simulink model "Reference_model_Control_Engineering"  (R2021b)
settings: Solver=FixedStepDiscrete  StartTime=0.0  StopTime=inf  FixedStep=Ts  RelTol=1e-3  EnableMultiTasking=on
InitFcn:
  | Fs = 4000; Ts = 1/Fs; tsim = 29.9997;
libraries: sperte_lib x116
settings Model: SimulationMode=external  Creator=Enzo  LastModifiedBy=20191981
settings SolverCC: AlgebraicLoopSolver=TrustRegion  PositivePriorityOrder=on
settings DataIOCC: SaveOutput=off  DSMLogging=off  SaveTime=off  ReturnWorkspaceOutputs=off
settings OptimizationCC: EnhancedBackFolding=on  PassReuseOutputArgsThreshold=0  MaxStackSize=64  OptimizeBlockOrder=speed  DifferentSizesBufferReuse=on  OptimizationCustomize=off
settings DebuggingCC: ParameterTunabilityLossMsg=error  SFMachineParentedDataDiag=warning  ArithmeticOperatorsInVariantConditions=warning
settings HardwareCC: ProdBitPerPointer=32  ProdBitPerSizeT=32  ProdBitPerPtrDiffT=32  ProdLargestAtomicInteger=Long  ProdLargestAtomicFloat=Double  ProdWordSize=32  ProdLongLongMode=on  ProdHWDeviceType=ARM Compatible->ARM Cortex  UseEmbeddedCoderFeatures=off
settings SFSimCC: CustomCodeUndefinedFunction=UseInterfaceOnly
settings RTWCC: Description=Embedded Coder  SystemTargetFile=ert.tlc  HardwareBoard=Raspberry Pi  TLCOptions="-aInlineSetEventsForThisBaseRateFcn=TLC_FALSE -aSuppressMultiTaskScheduler=TLC_FALSE  -aRateBasedStepFcn=0"  TemplateMakefile=ert_default_tmf  PostCodeGenCommand="if (~verLessThan('matlab', '9.11')) codertarget.postCodeGenHookCommand(h);  SPERTE_postGenFunc(modelName, buildInfo); else; SPERTE_postGenFunc(h, buildInfo); end"  Toolchain=GNU GCC Embedded Linux  BuildConfiguration=Faster Runs
settings CodeAppCC: ForceParamTrailComments=on  OperatorAnnotations=on
settings ERTTargetCC: ERTCustomFileBanners=off  SupportContinuousTime=on  SupportNonInlinedSFcns=on  RemoveResetFunc=off  SupportVariableSizeSignals=on  ModelStepFunctionPrototypeControlCompliant=off  ExtMode=on  ExtModeMexArgs='sperte0.bwk.tue.nl' 0 17725  ERTSrcFileBannerTemplate=codertarget_code_template.cgt  ERTHdrFileBannerTemplate=codertarget_code_template.cgt  ERTDataSrcFileTemplate=codertarget_code_template.cgt  ERTDataHdrFileTemplate=codertarget_code_template.cgt

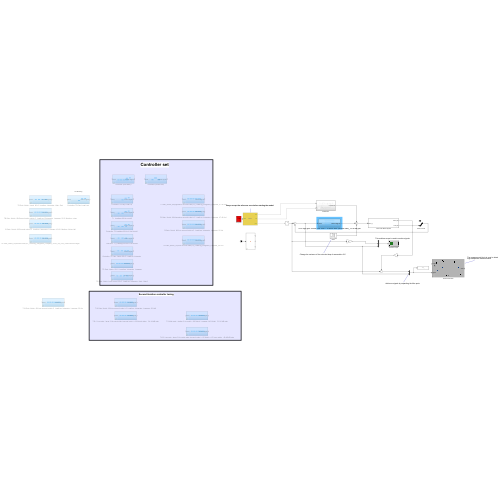
[thumbnail: Simulink's stored preview of the top-level diagram]
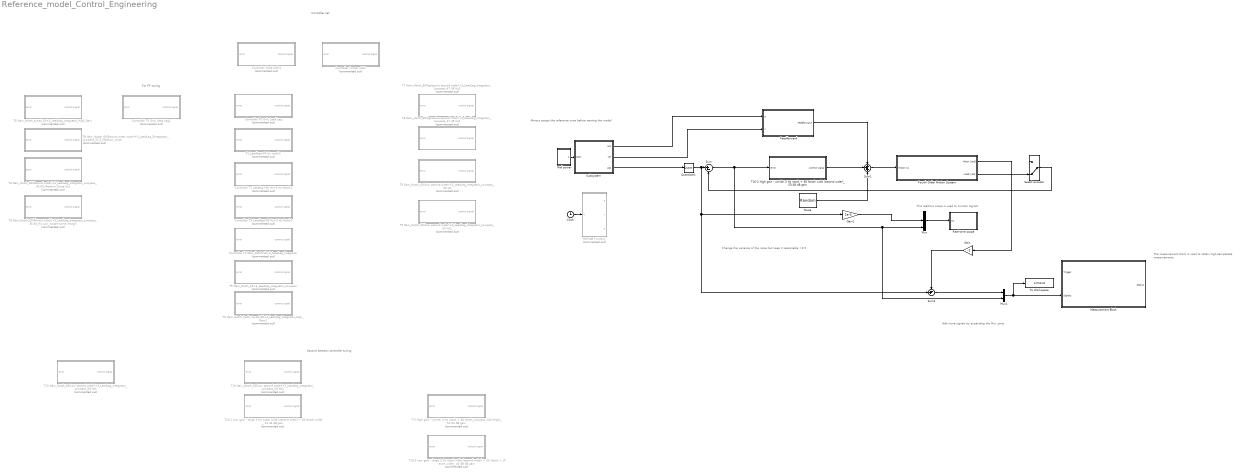
== system Reference_model_Control_Engineering ==
  note: Add more signals by expanding the Mux ports
  note: The measurement block is used to obtain high-samplerate measurements
  note: This realtime scope is used to monitor signals
  note: Always accept the reference once before starting the model.
  note: Change the variance of the noise but keep it reasonable <0.5
  note: Second iteration controller tuning
  note: For FF tuning
  note: Controller set
  Clock : Clock
  Controller (load side)1 : Subsystem  Commented=on
  Controller (motor side) : Subsystem  Commented=on
  Controller T0 Only Lead Lag : Subsystem  Commented=on
  Controller T0 Only Lead Lag1 : Subsystem  Commented=on
  Controller T2 Leadlag+60 Hz+3 Hz Notch1 : Subsystem  Commented=on
  Controller T3_Leadlag+60 Hz+3 Hz Notch1 : Subsystem  Commented=on
  Controller T4 Gain_Notch 60+3_LeadLag_Integrator : Subsystem  Commented=on
  Feedforward : Subsystem
  Fourth Order Motion System : Subsystem
  Gain : Gain  Gain=-1
  Gain1 : Gain  Gain=1e-3
  MATLAB Function : MATLAB Function  Commented=on  TreatAsAtomicUnit=on
  Measurement Block : Subsystem  Description=|  Priority=-1  mask(SPERTE Lib){N_samples=300000, triggertype=2, trigger_command=0}
      | Perform on-demand measurements to file using this block.
      | 
      | It can be used in 2 ways:
      | 1) Set the mask triggertype parameter to manual and use the trigger input signal to trigger a measurement.
      | You can do this by providing a 0 to 1 transition.
      | Keep it low after you start/complete the measurement, or it will measure again.
      | A file is created with measurement_0,1,2... etc
      | 
      | 2) Keep the model running, and trigger a measurement from the commandline or Matlab script.
      | For example:
      | 
      | % How many samples to measure?
      | N_samples = Fs*5;
      | % Do the measurement
      | SPERTE_Perform_Measurement(N_samples);
      | % Get the latest file
      | file_list = SPERTE_Get_Latest_Measurement(p,1,'./data');
      | % How many signals did you record?
      | N_signals = 3;
      | % Convert the .bin to .mat and return the results
      | measurement = SPERTE_Bin_To_Mat(file_list,N_signals);
      mask prompts: N_samples "Number of samples"; trigger_command "Trigger command"
      mask help:
      | This block implements a measurement to file sink.
      | It can be used in two ways:
      | 1) Triggered from the simulink model
      | 2) Triggered from the command line
      mask Help:
      | Perform on-demand measurements to file using this block.
      | 
      | It can be used in 2 ways:
      | 1) Set the mask triggertype parameter to manual and use the trigger input signal to trigger a measurement.
      | You can do this by providing a 0 to 1 transition.
      | Keep it low after you start/complete the measurement, or it will measure again.
      | A file is created with measurement_0,1,2... etc
      | 
      | 2) Keep the model running, and trigger a measurement from the commandline or Matlab script.
      | For example:
      | 
      | % How many samples to measure?
      | N_samples = Fs*5;
      | % Do the measurement
      | SPERTE_Perform_Measurement(N_samples);
      | % Get the latest file
      | file_list = SPERTE_Get_Latest_Measurement(p,1,'./data');
      | % How many signals did you record?
      | N_signals = 3;
      | % Convert the .bin to .mat and return the results
      | measurement = SPERTE_Bin_To_Mat(file_list,N_signals);
      mask TypeOptions N_samples: SPERTE_measurement_samples/Value
      mask TypeOptions trigger_command: SPERTE_measurement_trigger_command/Value
      mask DialogControl BlockName Prompt: Sperte measurement block.
      mask DialogControl Desc Prompt: Can be used to trace signals to .bin file on the Raspberry Pi.  Can be triggered through signals in the simulink model or manually.
      mask DialogControl TriggerText Prompt: Manual (0), Command (1), Both (2)
      mask Display: ud = get_param(gcb,'UserData');image(ud.x);
  Mux : Mux  Inputs=3
  Mux1 : Mux  Inputs=2
  Noise : RandomNumber  Variance=0  SampleTime=Ts
  Quantizer1 : Quantizer  QuantizationInterval=(2*pi)/(500*4)
  Real-time scope : Subsystem  Priority=0  mask(Scope){Sample_Time=1/500}
      mask prompts: Sample_Time "Scope sample time"
      mask help:
      | Realtime Scope block allows one to view the signals while the model is running.
      | The signals are downsampled to a specified sample rate (in the mask parameter) to reduce communication overhead.
      settings: CopyFcn=set_param(gcb,'LinkStatus','None')  OpenFcn=open_system(strcat(get_param(gcb,'Parent'),'/',get_param(gcb,'Name'),'/Live_Scope'),'force');
      mask TypeOptions Sample_Time: Downsample/OutPortSampleTime
      mask DialogControl scopebutton Prompt: Open the live scope
      mask DialogControl scopebutton Callback: open_system(strcat(get_param(gcb,'Parent'),'/',get_param(gcb,'Name'),'/Live_Scope'));
      mask Display: ud = get_param(gcb,'UserData');image(ud.x);
  Ref power : Subsystem  mask(On/Off Switch){stat=On}
      mask prompts: stat "Switch"
      mask TypeOptions stat: On | Off
  Select encoder : ManualSwitch  CurrentSetting=0
  Subsystem : Subsystem  mask(Ref3){}
      settings: OpenFcn=global ref_part; cb_axes 1
      mask Display: disp('Ref3');
  Sum : Sum  Inputs=|+-
  Sum1 : Sum  Inputs=+++
  Sum2 : Sum  Inputs=-+|
  T-II High gain - similar 3 Hz notch + 60 Notch_Lowpass 140 (High)_ 51.04 dB gain : Subsystem  Commented=on
  T10 Gain_Notch_60(Low second order)+3_LeadLag_Integrator_Lowpass_50 Hz1 : Subsystem  Commented=on
  T10 Gain_Notch_60(Low second order)+3_LeadLag_Integrator_Lowpass_50 Hz2 : Subsystem  Commented=on
  T10-1 Low gain - large 3 Hz notch wide (second order) + 60 Notch wider _ 24.44 dB gain : Subsystem  Commented=on
  T10-2 High gain - similar 3 Hz notch + 60 Notch wide (second order)_ 53.68 dB gain : Subsystem
  T10-3 Low gain - large 3 Hz notch wide (second order) + 60 Notch + LP even wider_ 40 dB dB gain : Subsystem  Commented=on
  T1_Leadlag+60 Hz notch2 : Subsystem  Commented=on
  T5 Gain_Notch_60+3_LeadLag_Integrator_Lowpass : Subsystem  Commented=on
  T5 Gain_Notch_tuned_60+3_LeadLag_Integrator_High_Gain : Subsystem  Commented=on
  T6 Gain_Notch_badly tuned_60+3_LeadLag_Integrator_High_Gain2 : Subsystem  Commented=on
  T7 Gain_Notch_60(Agressive second order)+3_LeadLag_Integrator_Lowpass_47.49 Hz2 : Subsystem  Commented=on
  T8 Gain_Notch_60(Agressive second order)+3_LeadLag_Integrator_Lowpass_47.49 Hz1 : Subsystem  Commented=on
  T8 Gain_Notch_60(Almost notch)+3_LeadLag_Integrator_Lowpass_35.60_Hz_Low_noise+some margin : Subsystem  Commented=on
  T9 Gain_Notch_60(Low second order)+3_LeadLag_Integrator_Lowpass_50 Hz : Subsystem  Commented=on
  T9 Gain_Notch_60(Low second order)+3_LeadLag_Integrator_Lowpass_50 Hz1 : Subsystem  Commented=on
  TA Gain_Notch_60(Second order)+3_LeadLag_Integrator_Lowpass_43.69_Medium_Noise Hz1 : Subsystem  Commented=on
  TB Gain_Notch_60(Second order notch)+3_LeadLag_DIntegrator_Lowpass_52.5_Medium_noise : Subsystem  Commented=on
  To Workspace : ToWorkspace  VariableName=simout  SampleTime=-1
  wires:
  Select encoder/1 -> Sum/2
  Sum1/1 -> Fourth Order Motion System/1(Motor [v])
  Sum/1 -> T10-2 High gain - similar 3 Hz notch + 60 Notch wide (second order)_ 53.68 dB gain/1(error), Mux1/2, Mux/3
  Quantizer1/1 -> Sum2/2, Gain1/1, Sum/1
  Ref power/1(On/Off) -> Subsystem/1(start)
  Mux/1 -> Real-time scope/1(In1)
  Noise/1 -> Sum1/3
  Mux1/1 -> To Workspace/1, Measurement Block/2(Signals)
  Clock/1 -> MATLAB Function/1(t)
  Feedforward/1(Feedforward) -> Sum1/1
  Gain/1 -> Sum2/1
  Subsystem/3(pos) -> Quantizer1/1
  Subsystem/2(vel) -> Feedforward/2(v)
  Subsystem/1(acc) -> Feedforward/1(a)
  Fourth Order Motion System/2(Load [rad]) -> Select encoder/2
  Fourth Order Motion System/1(Motor [rad]) -> Gain/1
  T10-2 High gain - similar 3 Hz notch + 60 Notch wide (second order)_ 53.68 dB gain/1(control signal) -> Sum1/2
  Gain1/1 -> Mux/2
  Sum2/1 -> Mux1/1

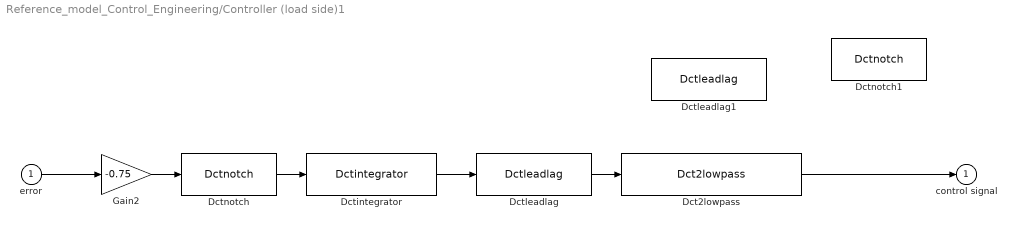
== system Reference_model_Control_Engineering/Controller (load side)1 ==
  error : Inport
  Dct2lowpass : sperte_lib/Dct2lowpass  f_den=60  b_den=0.075
      settings: SourceProductName=SPERTE project library
  Dctintegrator : sperte_lib/Dctintegrator  f_num=7.5
      settings: SourceProductName=SPERTE project library
  Dctleadlag : sperte_lib/Dctleadlag  f_num=4.5  f_den=1000
      settings: SourceProductName=SPERTE project library
  Dctleadlag1 : sperte_lib/Dctleadlag  f_num=5  f_den=50
      settings: SourceProductName=SPERTE project library
  Dctnotch : sperte_lib/Dctnotch  f_num=60.9  b_num=0.015  f_den=95  b_den=0.90
      settings: SourceProductName=SPERTE project library
  Dctnotch1 : sperte_lib/Dctnotch  f_num=2.6  b_num=0.3  f_den=2.6  b_den=0.001
      settings: SourceProductName=SPERTE project library
  Gain2 : Gain  Gain=-0.75
  control signal : Outport
  wires:
  error/1 -> Gain2/1
  Gain2/1 -> Dctnotch/1
  Dctnotch/1 -> Dctintegrator/1
  Dctintegrator/1 -> Dctleadlag/1
  Dctleadlag/1 -> Dct2lowpass/1
  Dct2lowpass/1 -> control signal/1

== system Reference_model_Control_Engineering/Controller (motor side) ==
  error : Inport
  Dctintegrator : sperte_lib/Dctintegrator  f_num=5
      settings: SourceProductName=SPERTE project library
  Dctleadlag : sperte_lib/Dctleadlag  f_num=6  f_den=130
      settings: SourceProductName=SPERTE project library
  Dctnotch : sperte_lib/Dctnotch  f_num=59  b_num=0.05  f_den=63  b_den=0.5
      settings: SourceProductName=SPERTE project library
  Gain2 : Gain  Gain=4.06
  control signal : Outport
  wires:
  error/1 -> Gain2/1
  Dctleadlag/1 -> control signal/1
  Gain2/1 -> Dctnotch/1
  Dctnotch/1 -> Dctleadlag/1

== system Reference_model_Control_Engineering/Controller T0 Only Lead Lag ==
  error : Inport
  Dctleadlag1 : sperte_lib/Dctleadlag  f_num=5  f_den=50
      settings: SourceProductName=SPERTE project library
  Dctnotch1 : sperte_lib/Dctnotch  f_num=2.6  b_num=0.3  f_den=2.6  b_den=0.001
      settings: SourceProductName=SPERTE project library
  Gain2 : Gain  Gain=-1
  Test_0_Dctleadlag : sperte_lib/Dctleadlag  f_num=6  f_den=17
      settings: SourceProductName=SPERTE project library
  control signal : Outport
  wires:
  error/1 -> Gain2/1
  Test_0_Dctleadlag/1 -> control signal/1
  Gain2/1 -> Test_0_Dctleadlag/1

== system Reference_model_Control_Engineering/Controller T0 Only Lead Lag1 ==
  error : Inport
  Dctleadlag1 : sperte_lib/Dctleadlag  f_num=5  f_den=50
      settings: SourceProductName=SPERTE project library
  Dctnotch1 : sperte_lib/Dctnotch  f_num=2.6  b_num=0.3  f_den=2.6  b_den=0.001
      settings: SourceProductName=SPERTE project library
  Gain2 : Gain  Gain=-1
  Test_0_Dctleadlag : sperte_lib/Dctleadlag  f_num=6  f_den=17
      settings: SourceProductName=SPERTE project library
  control signal : Outport
  wires:
  error/1 -> Gain2/1
  Test_0_Dctleadlag/1 -> control signal/1
  Gain2/1 -> Test_0_Dctleadlag/1

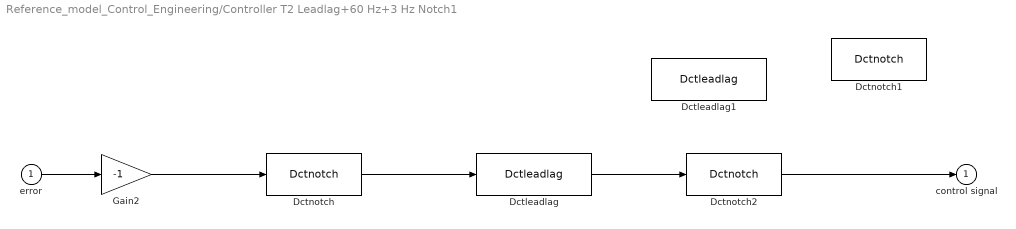
== system Reference_model_Control_Engineering/Controller T2 Leadlag+60 Hz+3 Hz Notch1 ==
  error : Inport
  Dctleadlag : sperte_lib/Dctleadlag  f_num=4.4195  f_den=180
      settings: SourceProductName=SPERTE project library
  Dctleadlag1 : sperte_lib/Dctleadlag  f_num=5  f_den=50
      settings: SourceProductName=SPERTE project library
  Dctnotch : sperte_lib/Dctnotch  f_num=60.95  b_num=0.01  f_den=60.95  b_den=0.6
      settings: SourceProductName=SPERTE project library
  Dctnotch1 : sperte_lib/Dctnotch  f_num=2.6  b_num=0.3  f_den=2.6  b_den=0.001
      settings: SourceProductName=SPERTE project library
  Dctnotch2 : sperte_lib/Dctnotch  f_num=3.25  b_num=0.5  f_den=3.25  b_den=0.025
      settings: SourceProductName=SPERTE project library
  Gain2 : Gain  Gain=-1
  control signal : Outport
  wires:
  error/1 -> Gain2/1
  Gain2/1 -> Dctnotch/1
  Dctleadlag/1 -> Dctnotch2/1
  Dctnotch/1 -> Dctleadlag/1
  Dctnotch2/1 -> control signal/1

== system Reference_model_Control_Engineering/Controller T3_Leadlag+60 Hz+3 Hz Notch1 ==
  error : Inport
  Dctleadlag : sperte_lib/Dctleadlag  f_num=5  f_den=400
      settings: SourceProductName=SPERTE project library
  Dctnotch : sperte_lib/Dctnotch  f_num=60.6  b_num=0.015  f_den=60.6  b_den=0.5
      settings: SourceProductName=SPERTE project library
  Dctnotch2 : sperte_lib/Dctnotch  f_num=3.25  b_num=0.5  f_den=3.25  b_den=0.025
      settings: SourceProductName=SPERTE project library
  Gain2 : Gain  Gain=-0.95
  control signal : Outport
  wires:
  error/1 -> Gain2/1
  Gain2/1 -> Dctnotch/1
  Dctleadlag/1 -> Dctnotch2/1
  Dctnotch/1 -> Dctleadlag/1
  Dctnotch2/1 -> control signal/1

== system Reference_model_Control_Engineering/Controller T4 Gain_Notch 60+3_LeadLag_Integrator ==
  error : Inport
  Dctintegrator : sperte_lib/Dctintegrator  f_num=7
      settings: SourceProductName=SPERTE project library
  Dctleadlag : sperte_lib/Dctleadlag  f_num=3.975  f_den=400
      settings: SourceProductName=SPERTE project library
  Dctnotch : sperte_lib/Dctnotch  f_num=60.6  b_num=0.015  f_den=90  b_den=0.5
      settings: SourceProductName=SPERTE project library
  Dctnotch2 : sperte_lib/Dctnotch  f_num=3.25  b_num=0.5  f_den=3.25  b_den=0.025
      settings: SourceProductName=SPERTE project library
  Gain2 : Gain  Gain=-0.95
  control signal : Outport
  wires:
  error/1 -> Gain2/1
  Gain2/1 -> Dctnotch/1
  Dctleadlag/1 -> Dctnotch2/1
  Dctnotch/1 -> Dctleadlag/1
  Dctnotch2/1 -> Dctintegrator/1
  Dctintegrator/1 -> control signal/1

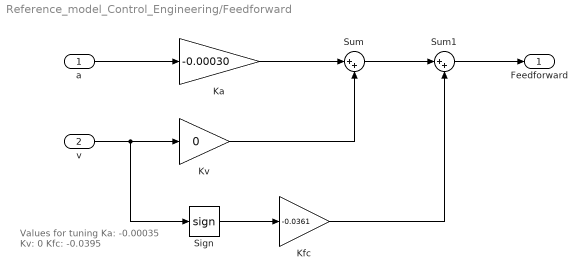
== system Reference_model_Control_Engineering/Feedforward ==
  note: Values for tuning
      | Ka: -0.00035
      | Kv: 	0
      | Kfc: -0.0395
  a : Inport
  v : Inport  Port=2
  Ka : Gain  Gain=-0.00030
  Kfc : Gain  Gain=-0.0361
  Kv : Gain  Gain=0
  Sign : Signum
  Sum : Sum  Inputs=|++
  Sum1 : Sum  Inputs=|++
  Feedforward : Outport
  wires:
  a/1 -> Ka/1
  Ka/1 -> Sum/1
  v/1 -> Sign/1, Kv/1
  Kv/1 -> Sum/2
  Sign/1 -> Kfc/1
  Sum/1 -> Sum1/1
  Kfc/1 -> Sum1/2
  Sum1/1 -> Feedforward/1

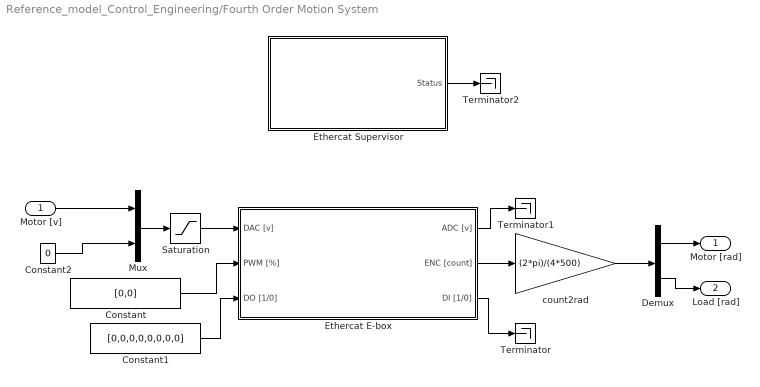
== system Reference_model_Control_Engineering/Fourth Order Motion System ==
  Motor [v] : Inport
  Constant : Constant  Value=[0,0]
  Constant1 : Constant  Value=[0,0,0,0,0,0,0,0]
  Constant2 : Constant  Value=0
  Demux : Demux  Outputs=2
  Ethercat E-box : Subsystem  Priority=-2  mask(Sperte Lib){link_id=0}
      mask prompts: link_id "Link ID of the specific ebox"
      mask help:
      | This block implements a single E-box device.
      | Ensure that if you have multiple E-box devices that they each have an unique link_id.
      |
      | You MUST have an Ethercat Initialize block in your model to be able to use this block.
      mask Display: ud = get_param(gcb,'UserData');image(ud.x);
  Ethercat Supervisor : Subsystem  Description=Must be executed first, keep at -1 priority (highest)  Priority=-3  mask(Sperte Lib){portid=0, ectimeout=500}
      mask prompts: portid "Ethernet port number for the Ethercat protocol (default 0 = eth0)"; ectimeout "Timeout of the Ethercat protocol in microseconds."
      mask help:
      | This block initializes the Ethercat connection on the Raspberry Pi.
      |
      | This enables you to use multiple E-box devices by including multiple blocks of the "Ethercat E-box" type.
      mask Display: ud = get_param(gcb,'UserData');image(ud.x);
  Mux : Mux  Inputs=2
  Saturation : Saturate  UpperLimit=2.5  LowerLimit=-2.5
  Terminator : Terminator
  Terminator1 : Terminator
  Terminator2 : Terminator
  count2rad : Gain  Gain=(2*pi)/(4*500)
  Motor [rad] : Outport
  Load [rad] : Outport  Port=2
  wires:
  Ethercat E-box/1(ADC [v]) -> Terminator1/1
  Ethercat E-box/2(ENC [count]) -> count2rad/1
  Constant/1 -> Ethercat E-box/2(PWM [%])
  Mux/1 -> Saturation/1
  count2rad/1 -> Demux/1
  Motor [v]/1 -> Mux/1
  Constant2/1 -> Mux/2
  Demux/1 -> Motor [rad]/1
  Demux/2 -> Load [rad]/1
  Ethercat E-box/3(DI [1/0]) -> Terminator/1
  Constant1/1 -> Ethercat E-box/3(DO [1/0])
  Saturation/1 -> Ethercat E-box/1(DAC [v])
  Ethercat Supervisor/1(Status) -> Terminator2/1

== system Reference_model_Control_Engineering/Measurement Block ==
  Trigger : Inport
  Signals : Inport  Port=2
  SPERTE_measurement_function : MATLAB Function  TreatAsAtomicUnit=on
  SPERTE_measurement_samples : Constant  Value=N_samples  OutDataTypeStr=uint32
  SPERTE_measurement_trigger_command : Constant  Value=trigger_command  OutDataTypeStr=uint8
  Status : Outport
  wires:
  SPERTE_measurement_samples/1 -> SPERTE_measurement_function/4(N_samples)
  SPERTE_measurement_trigger_command/1 -> SPERTE_measurement_function/3(trigger_command)
  Signals/1 -> SPERTE_measurement_function/1(u)
  Trigger/1 -> SPERTE_measurement_function/2(trigger_manual)
  SPERTE_measurement_function/1(status) -> Status/1

== system Reference_model_Control_Engineering/Real-time scope ==
  note: The default scope sample rate is 500 Hz.
      | This can be changed by right-click on the Realtime Scope block.
      | Then selecting -> Mask -> Mask parameters.
  In1 : Inport
  Buffer : SignalConversion  OverrideOpt=off
  Downsample : RateTransition  OutPortSampleTime=Sample_Time
  Live_Scope : Scope
  wires:
  In1/1 -> Buffer/1
  Downsample/1 -> Live_Scope/1
  Buffer/1 -> Downsample/1

== system Reference_model_Control_Engineering/Ref power ==
  Start setpoint : Constant  Value=stat
  On/Off : Outport
  wires:
  Start setpoint/1 -> On/Off/1

== system Reference_model_Control_Engineering/Subsystem ==
  start : Inport
  Demux : Demux  Outputs=3
      settings: DisplayOption=none
  S-Function : S-Function  FunctionName=ref3b  Parameters=ref_part  SFunctionDeploymentMode=off  EnableBusSupport=off
      settings: OpenFcn=global ref_part; r3g_main
  acc : Outport
  vel : Outport  Port=2
  pos : Outport  Port=3
  wires:
  S-Function/1 -> Demux/1
  Demux/1 -> acc/1
  Demux/2 -> vel/1
  Demux/3 -> pos/1
  start/1 -> S-Function/1

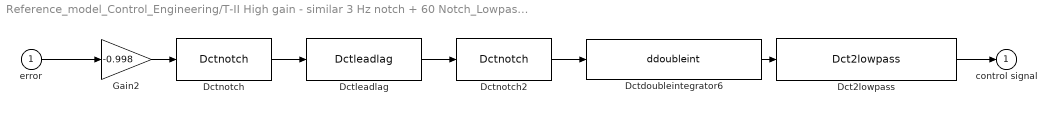
== system Reference_model_Control_Engineering/T-II High gain - similar 3 Hz notch + 60 Notch_Lowpass 140 (High)_ 51.04 dB gain ==
  error : Inport
  Dct2lowpass : sperte_lib/Dct2lowpass  f_den=140  b_den=0.5
      settings: SourceProductName=SPERTE project library
  Dctdoubleintegrator6 : S-Function  FunctionName=ddoubleint  Parameters=f_num, b_num, 0.001  SFunctionDeploymentMode=off  EnableBusSupport=off  mask(dctools){f_num=3.8, b_num=0.12}
      mask prompts: f_num "Zero [Hz]"; b_num "Damping [-]"
      mask help: This block implements a discrete time double-integrator filter with complex zero-pair.
      mask Display: disp('DCT double-integrator')
  Dctleadlag : sperte_lib/Dctleadlag  f_num=5.842  f_den=600
      settings: SourceProductName=SPERTE project library
  Dctnotch : sperte_lib/Dctnotch  f_num=60.6  b_num=0.001  f_den=70  b_den=0.6
      settings: SourceProductName=SPERTE project library
  Dctnotch2 : sperte_lib/Dctnotch  f_num=3.5  b_num=0.5  f_den=3.5  b_den=0.01
      settings: SourceProductName=SPERTE project library
  Gain2 : Gain  Gain=-0.998
  control signal : Outport
  wires:
  error/1 -> Gain2/1
  Gain2/1 -> Dctnotch/1
  Dctleadlag/1 -> Dctnotch2/1
  Dctnotch/1 -> Dctleadlag/1
  Dctnotch2/1 -> Dctdoubleintegrator6/1
  Dctdoubleintegrator6/1 -> Dct2lowpass/1
  Dct2lowpass/1 -> control signal/1

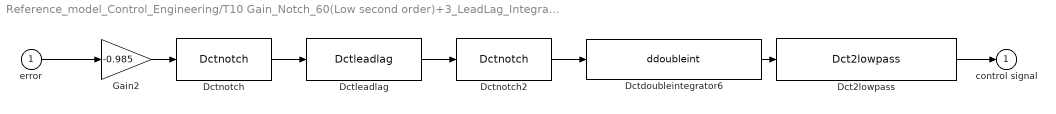
== system Reference_model_Control_Engineering/T10 Gain_Notch_60(Low second order)+3_LeadLag_Integrator_Lowpass_50 Hz1 ==
  error : Inport
  Dct2lowpass : sperte_lib/Dct2lowpass  f_den=140  b_den=0.5
      settings: SourceProductName=SPERTE project library
  Dctdoubleintegrator6 : S-Function  FunctionName=ddoubleint  Parameters=f_num, b_num, 0.001  SFunctionDeploymentMode=off  EnableBusSupport=off  mask(dctools){f_num=3.7, b_num=0.18}
      mask prompts: f_num "Zero [Hz]"; b_num "Damping [-]"
      mask help: This block implements a discrete time double-integrator filter with complex zero-pair.
      mask Display: disp('DCT double-integrator')
  Dctleadlag : sperte_lib/Dctleadlag  f_num=5.6  f_den=600
      settings: SourceProductName=SPERTE project library
  Dctnotch : sperte_lib/Dctnotch  f_num=60.6  b_num=0.001  f_den=80  b_den=0.7
      settings: SourceProductName=SPERTE project library
  Dctnotch2 : sperte_lib/Dctnotch  f_num=3.25  b_num=0.5  f_den=3.25  b_den=0.01
      settings: SourceProductName=SPERTE project library
  Gain2 : Gain  Gain=-0.985
  control signal : Outport
  wires:
  error/1 -> Gain2/1
  Gain2/1 -> Dctnotch/1
  Dctleadlag/1 -> Dctnotch2/1
  Dctnotch/1 -> Dctleadlag/1
  Dctnotch2/1 -> Dctdoubleintegrator6/1
  Dctdoubleintegrator6/1 -> Dct2lowpass/1
  Dct2lowpass/1 -> control signal/1

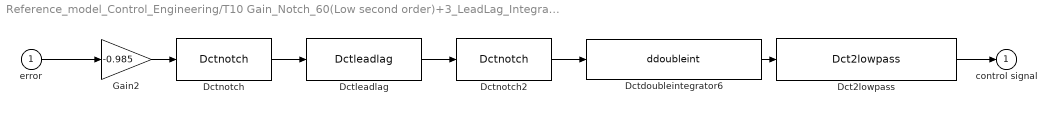
== system Reference_model_Control_Engineering/T10 Gain_Notch_60(Low second order)+3_LeadLag_Integrator_Lowpass_50 Hz2 ==
  error : Inport
  Dct2lowpass : sperte_lib/Dct2lowpass  f_den=140  b_den=0.5
      settings: SourceProductName=SPERTE project library
  Dctdoubleintegrator6 : S-Function  FunctionName=ddoubleint  Parameters=f_num, b_num, 0.001  SFunctionDeploymentMode=off  EnableBusSupport=off  mask(dctools){f_num=3.7, b_num=0.18}
      mask prompts: f_num "Zero [Hz]"; b_num "Damping [-]"
      mask help: This block implements a discrete time double-integrator filter with complex zero-pair.
      mask Display: disp('DCT double-integrator')
  Dctleadlag : sperte_lib/Dctleadlag  f_num=5.6  f_den=600
      settings: SourceProductName=SPERTE project library
  Dctnotch : sperte_lib/Dctnotch  f_num=60.6  b_num=0.001  f_den=80  b_den=0.7
      settings: SourceProductName=SPERTE project library
  Dctnotch2 : sperte_lib/Dctnotch  f_num=3.25  b_num=0.5  f_den=3.25  b_den=0.01
      settings: SourceProductName=SPERTE project library
  Gain2 : Gain  Gain=-0.985
  control signal : Outport
  wires:
  error/1 -> Gain2/1
  Gain2/1 -> Dctnotch/1
  Dctleadlag/1 -> Dctnotch2/1
  Dctnotch/1 -> Dctleadlag/1
  Dctnotch2/1 -> Dctdoubleintegrator6/1
  Dctdoubleintegrator6/1 -> Dct2lowpass/1
  Dct2lowpass/1 -> control signal/1

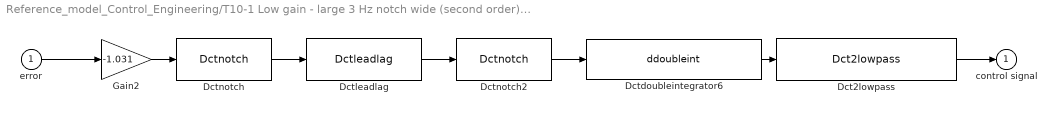
== system Reference_model_Control_Engineering/T10-1 Low gain - large 3 Hz notch wide (second order) + 60 Notch wider _ 24.44 dB gain ==
  error : Inport
  Dct2lowpass : sperte_lib/Dct2lowpass  f_den=120  b_den=0.5
      settings: SourceProductName=SPERTE project library
  Dctdoubleintegrator6 : S-Function  FunctionName=ddoubleint  Parameters=f_num, b_num, 0.001  SFunctionDeploymentMode=off  EnableBusSupport=off  mask(dctools){f_num=1.25, b_num=0.065}
      mask prompts: f_num "Zero [Hz]"; b_num "Damping [-]"
      mask help: This block implements a discrete time double-integrator filter with complex zero-pair.
      mask Display: disp('DCT double-integrator')
  Dctleadlag : sperte_lib/Dctleadlag  f_num=4.825  f_den=700
      settings: SourceProductName=SPERTE project library
  Dctnotch : sperte_lib/Dctnotch  f_num=60.6  b_num=0.005  f_den=82  b_den=0.85
      settings: SourceProductName=SPERTE project library
  Dctnotch2 : sperte_lib/Dctnotch  f_num=3.7  b_num=0.6  f_den=3.25  b_den=0.01
      settings: SourceProductName=SPERTE project library
  Gain2 : Gain  Gain=-1.031
  control signal : Outport
  wires:
  error/1 -> Gain2/1
  Gain2/1 -> Dctnotch/1
  Dctleadlag/1 -> Dctnotch2/1
  Dctnotch/1 -> Dctleadlag/1
  Dctnotch2/1 -> Dctdoubleintegrator6/1
  Dctdoubleintegrator6/1 -> Dct2lowpass/1
  Dct2lowpass/1 -> control signal/1

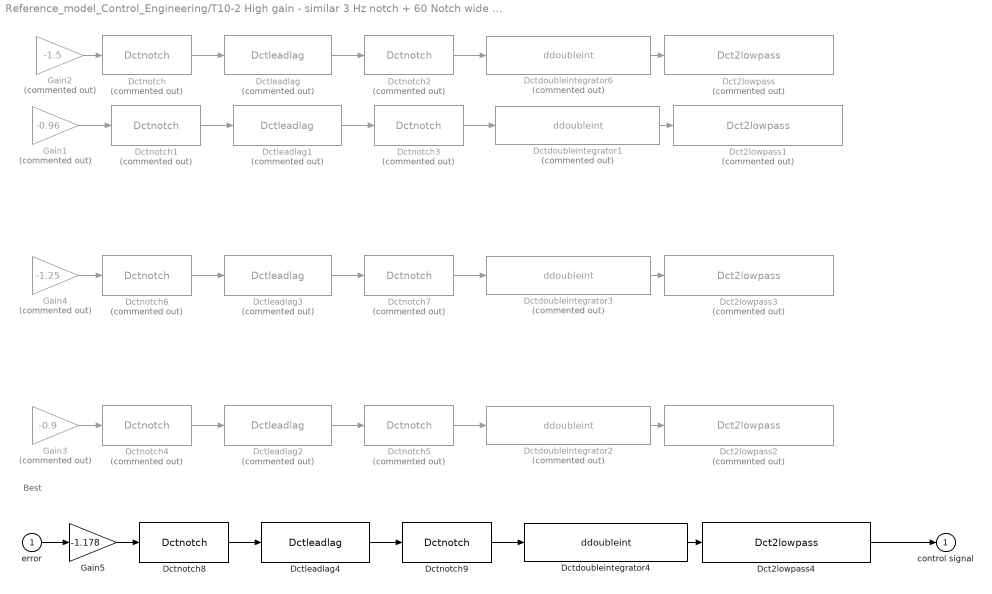
== system Reference_model_Control_Engineering/T10-2 High gain - similar 3 Hz notch + 60 Notch wide (second order)_ 53.68 dB gain ==
  note: Best
  error : Inport
  Dct2lowpass{,1..3} (4 alike) : sperte_lib/Dct2lowpass  Commented=on  f_den=120  b_den=0.5
      settings: SourceProductName=SPERTE project library
  Dct2lowpass4 : sperte_lib/Dct2lowpass  f_den=120  b_den=0.5
      settings: SourceProductName=SPERTE project library
  Dctdoubleintegrator1 : S-Function  Commented=on  FunctionName=ddoubleint  Parameters=f_num, b_num, 0.001  SFunctionDeploymentMode=off  EnableBusSupport=off  mask(dctools){f_num=1, b_num=0.5}
      mask prompts: f_num "Zero [Hz]"; b_num "Damping [-]"
      mask help: This block implements a discrete time double-integrator filter with complex zero-pair.
      mask Display: disp('DCT double-integrator')
  Dctdoubleintegrator2 : S-Function  Commented=on  FunctionName=ddoubleint  Parameters=f_num, b_num, 0.001  SFunctionDeploymentMode=off  EnableBusSupport=off  mask(dctools){f_num=4.2, b_num=0.25}
      mask prompts: f_num "Zero [Hz]"; b_num "Damping [-]"
      mask help: This block implements a discrete time double-integrator filter with complex zero-pair.
      mask Display: disp('DCT double-integrator')
  Dctdoubleintegrator3 : S-Function  Commented=on  FunctionName=ddoubleint  Parameters=f_num, b_num, 0.001  SFunctionDeploymentMode=off  EnableBusSupport=off  mask(dctools){f_num=4.5, b_num=0.25}
      mask prompts: f_num "Zero [Hz]"; b_num "Damping [-]"
      mask help: This block implements a discrete time double-integrator filter with complex zero-pair.
      mask Display: disp('DCT double-integrator')
  Dctdoubleintegrator4 : S-Function  FunctionName=ddoubleint  Parameters=f_num, b_num, 0.001  SFunctionDeploymentMode=off  EnableBusSupport=off  mask(dctools){f_num=4.5, b_num=0.25}
      mask prompts: f_num "Zero [Hz]"; b_num "Damping [-]"
      mask help: This block implements a discrete time double-integrator filter with complex zero-pair.
      mask Display: disp('DCT double-integrator')
  Dctdoubleintegrator6 : S-Function  Commented=on  FunctionName=ddoubleint  Parameters=f_num, b_num, 0.001  SFunctionDeploymentMode=off  EnableBusSupport=off  mask(dctools){f_num=1, b_num=0.5}
      mask prompts: f_num "Zero [Hz]"; b_num "Damping [-]"
      mask help: This block implements a discrete time double-integrator filter with complex zero-pair.
      mask Display: disp('DCT double-integrator')
  Dctleadlag : sperte_lib/Dctleadlag  Commented=on  f_num=4.1  f_den=600
      settings: SourceProductName=SPERTE project library
  Dctleadlag1 : sperte_lib/Dctleadlag  Commented=on  f_num=4.1  f_den=600
      settings: SourceProductName=SPERTE project library
  Dctleadlag2 : sperte_lib/Dctleadlag  Commented=on  f_num=5.055  f_den=600
      settings: SourceProductName=SPERTE project library
  Dctleadlag3 : sperte_lib/Dctleadlag  Commented=on  f_num=5.055  f_den=600
      settings: SourceProductName=SPERTE project library
  Dctleadlag4 : sperte_lib/Dctleadlag  f_num=5.055  f_den=600
      settings: SourceProductName=SPERTE project library
  Dctnotch : sperte_lib/Dctnotch  Commented=on  f_num=60.6  b_num=0.001  f_den=82  b_den=0.5
      settings: SourceProductName=SPERTE project library
  Dctnotch1 : sperte_lib/Dctnotch  Commented=on  f_num=60.6  b_num=0.001  f_den=82  b_den=0.5
      settings: SourceProductName=SPERTE project library
  Dctnotch2 : sperte_lib/Dctnotch  Commented=on  f_num=5  b_num=0.5  f_den=3.45  b_den=0.001
      settings: SourceProductName=SPERTE project library
  Dctnotch3 : sperte_lib/Dctnotch  Commented=on  f_num=3.75  b_num=0.5  f_den=3.5  b_den=0.001
      settings: SourceProductName=SPERTE project library
  Dctnotch4 : sperte_lib/Dctnotch  Commented=on  f_num=60.6  b_num=0.001  f_den=75  b_den=0.5
      settings: SourceProductName=SPERTE project library
  Dctnotch5 : sperte_lib/Dctnotch  Commented=on  f_num=3.5  b_num=0.4  f_den=3.5  b_den=0.001
      settings: SourceProductName=SPERTE project library
  Dctnotch6 : sperte_lib/Dctnotch  Commented=on  f_num=60.6  b_num=0.001  f_den=75  b_den=0.5
      settings: SourceProductName=SPERTE project library
  Dctnotch7 : sperte_lib/Dctnotch  Commented=on  f_num=3.75  b_num=0.45  f_den=3.5  b_den=0.001
      settings: SourceProductName=SPERTE project library
  Dctnotch8 : sperte_lib/Dctnotch  f_num=60.6  b_num=0.001  f_den=75  b_den=0.5
      settings: SourceProductName=SPERTE project library
  Dctnotch9 : sperte_lib/Dctnotch  f_num=3.9  b_num=0.4  f_den=3.5  b_den=0.001
      settings: SourceProductName=SPERTE project library
  Gain1 : Gain  Commented=on  Gain=-0.96
  Gain2 : Gain  Commented=on  Gain=-1.5
  Gain3 : Gain  Commented=on  Gain=-0.9
  Gain4 : Gain  Commented=on  Gain=-1.25
  Gain5 : Gain  Gain=-1.178
  control signal : Outport
  wires:
  Dctleadlag/1 -> Dctnotch2/1
  Dctnotch/1 -> Dctleadlag/1
  Dctnotch2/1 -> Dctdoubleintegrator6/1
  Dctdoubleintegrator6/1 -> Dct2lowpass/1
  Gain2/1 -> Dctnotch/1
  Dct2lowpass4/1 -> control signal/1
  Dctnotch1/1 -> Dctleadlag1/1
  Dctnotch3/1 -> Dctdoubleintegrator1/1
  Gain1/1 -> Dctnotch1/1
  Dctdoubleintegrator1/1 -> Dct2lowpass1/1
  Dctleadlag1/1 -> Dctnotch3/1
  error/1 -> Gain5/1
  Dctnotch7/1 -> Dctdoubleintegrator3/1
  Gain4/1 -> Dctnotch6/1
  Dctdoubleintegrator3/1 -> Dct2lowpass3/1
  Dctleadlag3/1 -> Dctnotch7/1
  Dctnotch6/1 -> Dctleadlag3/1
  Dctnotch5/1 -> Dctdoubleintegrator2/1
  Gain3/1 -> Dctnotch4/1
  Dctdoubleintegrator2/1 -> Dct2lowpass2/1
  Dctleadlag2/1 -> Dctnotch5/1
  Dctnotch4/1 -> Dctleadlag2/1
  Dctnotch8/1 -> Dctleadlag4/1
  Dctleadlag4/1 -> Dctnotch9/1
  Dctdoubleintegrator4/1 -> Dct2lowpass4/1
  Dctnotch9/1 -> Dctdoubleintegrator4/1
  Gain5/1 -> Dctnotch8/1

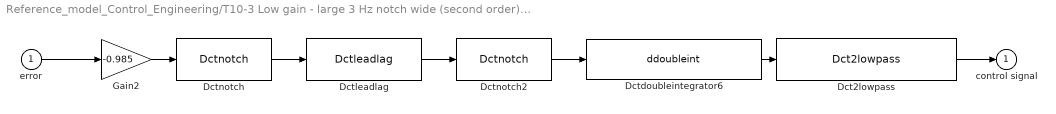
== system Reference_model_Control_Engineering/T10-3 Low gain - large 3 Hz notch wide (second order) + 60 Notch + LP even wider_ 40 dB dB gain ==
  error : Inport
  Dct2lowpass : sperte_lib/Dct2lowpass  f_den=140  b_den=0.5
      settings: SourceProductName=SPERTE project library
  Dctdoubleintegrator6 : S-Function  FunctionName=ddoubleint  Parameters=f_num, b_num, 0.001  SFunctionDeploymentMode=off  EnableBusSupport=off  mask(dctools){f_num=3.7, b_num=0.18}
      mask prompts: f_num "Zero [Hz]"; b_num "Damping [-]"
      mask help: This block implements a discrete time double-integrator filter with complex zero-pair.
      mask Display: disp('DCT double-integrator')
  Dctleadlag : sperte_lib/Dctleadlag  f_num=5.6  f_den=600
      settings: SourceProductName=SPERTE project library
  Dctnotch : sperte_lib/Dctnotch  f_num=60.6  b_num=0.001  f_den=80  b_den=0.7
      settings: SourceProductName=SPERTE project library
  Dctnotch2 : sperte_lib/Dctnotch  f_num=3.25  b_num=0.5  f_den=3.25  b_den=0.01
      settings: SourceProductName=SPERTE project library
  Gain2 : Gain  Gain=-0.985
  control signal : Outport
  wires:
  error/1 -> Gain2/1
  Gain2/1 -> Dctnotch/1
  Dctleadlag/1 -> Dctnotch2/1
  Dctnotch/1 -> Dctleadlag/1
  Dctnotch2/1 -> Dctdoubleintegrator6/1
  Dctdoubleintegrator6/1 -> Dct2lowpass/1
  Dct2lowpass/1 -> control signal/1

== system Reference_model_Control_Engineering/T1_Leadlag+60 Hz notch2 ==
  error : Inport
  Dctleadlag : sperte_lib/Dctleadlag  f_num=4.1  f_den=80
      settings: SourceProductName=SPERTE project library
  Dctleadlag1 : sperte_lib/Dctleadlag  f_num=5  f_den=50
      settings: SourceProductName=SPERTE project library
  Dctnotch : sperte_lib/Dctnotch  f_num=60.95  b_num=0.015  f_den=60.95  b_den=0.6
      settings: SourceProductName=SPERTE project library
  Dctnotch1 : sperte_lib/Dctnotch  f_num=2.6  b_num=0.3  f_den=2.6  b_den=0.001
      settings: SourceProductName=SPERTE project library
  Gain2 : Gain  Gain=-1
  control signal : Outport
  wires:
  error/1 -> Gain2/1
  Gain2/1 -> Dctnotch/1
  Dctleadlag/1 -> control signal/1
  Dctnotch/1 -> Dctleadlag/1

== system Reference_model_Control_Engineering/T5 Gain_Notch_60+3_LeadLag_Integrator_Lowpass ==
  error : Inport
  Dct2lowpass : sperte_lib/Dct2lowpass  f_den=100  b_den=0.1
      settings: SourceProductName=SPERTE project library
  Dctintegrator : sperte_lib/Dctintegrator  f_num=8
      settings: SourceProductName=SPERTE project library
  Dctleadlag : sperte_lib/Dctleadlag  f_num=3.975  f_den=400
      settings: SourceProductName=SPERTE project library
  Dctnotch : sperte_lib/Dctnotch  f_num=60.6  b_num=0.015  f_den=100  b_den=0.5
      settings: SourceProductName=SPERTE project library
  Dctnotch2 : sperte_lib/Dctnotch  f_num=3.25  b_num=0.5  f_den=3.25  b_den=0.025
      settings: SourceProductName=SPERTE project library
  Gain2 : Gain  Gain=-1.0079
  control signal : Outport
  wires:
  error/1 -> Gain2/1
  Gain2/1 -> Dctnotch/1
  Dctleadlag/1 -> Dctnotch2/1
  Dctnotch/1 -> Dctleadlag/1
  Dctnotch2/1 -> Dctintegrator/1
  Dctintegrator/1 -> Dct2lowpass/1
  Dct2lowpass/1 -> control signal/1

== system Reference_model_Control_Engineering/T5 Gain_Notch_tuned_60+3_LeadLag_Integrator_High_Gain ==
  error : Inport
  Dctintegrator : sperte_lib/Dctintegrator  f_num=2
      settings: SourceProductName=SPERTE project library
  Dctleadlag : sperte_lib/Dctleadlag  f_num=6  f_den=500
      settings: SourceProductName=SPERTE project library
  Dctnotch : sperte_lib/Dctnotch  f_num=60  b_num=0.001  f_den=70  b_den=0.5
      settings: SourceProductName=SPERTE project library
  Dctnotch2 : sperte_lib/Dctnotch  f_num=3.25  b_num=0.6  f_den=3.25  b_den=0.1
      settings: SourceProductName=SPERTE project library
  Gain2 : Gain  Gain=-1
  control signal : Outport
  wires:
  error/1 -> Gain2/1
  Gain2/1 -> Dctnotch/1
  Dctleadlag/1 -> Dctnotch2/1
  Dctnotch/1 -> Dctleadlag/1
  Dctnotch2/1 -> Dctintegrator/1
  Dctintegrator/1 -> control signal/1

== system Reference_model_Control_Engineering/T6 Gain_Notch_badly tuned_60+3_LeadLag_Integrator_High_Gain2 ==
  note: Moved the notch up to the right
  error : Inport
  Dctintegrator : sperte_lib/Dctintegrator  f_num=9
      settings: SourceProductName=SPERTE project library
  Dctleadlag : sperte_lib/Dctleadlag  f_num=3.975  f_den=400
      settings: SourceProductName=SPERTE project library
  Dctnotch : sperte_lib/Dctnotch  f_num=60.6  b_num=0.015  f_den=120  b_den=0.49
      settings: SourceProductName=SPERTE project library
  Dctnotch2 : sperte_lib/Dctnotch  f_num=3.25  b_num=0.5  f_den=3.25  b_den=0.025
      settings: SourceProductName=SPERTE project library
  Gain2 : Gain  Gain=-1.0079
  control signal : Outport
  wires:
  error/1 -> Gain2/1
  Gain2/1 -> Dctnotch/1
  Dctleadlag/1 -> Dctnotch2/1
  Dctnotch/1 -> Dctleadlag/1
  Dctnotch2/1 -> Dctintegrator/1
  Dctintegrator/1 -> control signal/1

== system Reference_model_Control_Engineering/T7 Gain_Notch_60(Agressive second order)+3_LeadLag_Integrator_Lowpass_47.49 Hz2 ==
  error : Inport
  Dct2lowpass : sperte_lib/Dct2lowpass  f_den=130  b_den=0.5
      settings: SourceProductName=SPERTE project library
  Dctintegrator : sperte_lib/Dctintegrator  f_num=8.25
      settings: SourceProductName=SPERTE project library
  Dctleadlag : sperte_lib/Dctleadlag  f_num=3.975  f_den=575
      settings: SourceProductName=SPERTE project library
  Dctnotch : sperte_lib/Dctnotch  f_num=60.6  b_num=0.001  f_den=400  b_den=0.45
      settings: SourceProductName=SPERTE project library
  Dctnotch2 : sperte_lib/Dctnotch  f_num=3.25  b_num=0.5  f_den=3.25  b_den=0.11
      settings: SourceProductName=SPERTE project library
  Gain2 : Gain  Gain=-1.024
  control signal : Outport
  wires:
  error/1 -> Gain2/1
  Gain2/1 -> Dctnotch/1
  Dctleadlag/1 -> Dctnotch2/1
  Dctnotch/1 -> Dctleadlag/1
  Dctnotch2/1 -> Dctintegrator/1
  Dctintegrator/1 -> Dct2lowpass/1
  Dct2lowpass/1 -> control signal/1

== system Reference_model_Control_Engineering/T8 Gain_Notch_60(Agressive second order)+3_LeadLag_Integrator_Lowpass_47.49 Hz1 ==
  error : Inport
  Dct2lowpass : sperte_lib/Dct2lowpass  f_den=130  b_den=0.5
      settings: SourceProductName=SPERTE project library
  Dctintegrator : sperte_lib/Dctintegrator  f_num=8.25
      settings: SourceProductName=SPERTE project library
  Dctleadlag : sperte_lib/Dctleadlag  f_num=3.975  f_den=575
      settings: SourceProductName=SPERTE project library
  Dctnotch : sperte_lib/Dctnotch  f_num=60.6  b_num=0.001  f_den=400  b_den=0.45
      settings: SourceProductName=SPERTE project library
  Dctnotch2 : sperte_lib/Dctnotch  f_num=3.25  b_num=0.5  f_den=3.25  b_den=0.11
      settings: SourceProductName=SPERTE project library
  Gain2 : Gain  Gain=-1.024
  control signal : Outport
  wires:
  error/1 -> Gain2/1
  Gain2/1 -> Dctnotch/1
  Dctleadlag/1 -> Dctnotch2/1
  Dctnotch/1 -> Dctleadlag/1
  Dctnotch2/1 -> Dctintegrator/1
  Dctintegrator/1 -> Dct2lowpass/1
  Dct2lowpass/1 -> control signal/1

== system Reference_model_Control_Engineering/T8 Gain_Notch_60(Almost notch)+3_LeadLag_Integrator_Lowpass_35.60_Hz_Low_noise+some margin ==
  error : Inport
  Dct2lowpass : sperte_lib/Dct2lowpass  f_den=120  b_den=0.5
      settings: SourceProductName=SPERTE project library
  Dctintegrator : sperte_lib/Dctintegrator  f_num=1.8
      settings: SourceProductName=SPERTE project library
  Dctleadlag : sperte_lib/Dctleadlag  f_num=6.21  f_den=500
      settings: SourceProductName=SPERTE project library
  Dctnotch : sperte_lib/Dctnotch  f_num=60.6  b_num=0.015  f_den=75  b_den=0.45
      settings: SourceProductName=SPERTE project library
  Dctnotch2 : sperte_lib/Dctnotch  f_num=3.25  b_num=0.5  f_den=3.25  b_den=0.025
      settings: SourceProductName=SPERTE project library
  Gain2 : Gain  Gain=-1.0029
  control signal : Outport
  wires:
  error/1 -> Gain2/1
  Gain2/1 -> Dctnotch/1
  Dctleadlag/1 -> Dctnotch2/1
  Dctnotch/1 -> Dctleadlag/1
  Dctnotch2/1 -> Dctintegrator/1
  Dctintegrator/1 -> Dct2lowpass/1
  Dct2lowpass/1 -> control signal/1

== system Reference_model_Control_Engineering/T9 Gain_Notch_60(Low second order)+3_LeadLag_Integrator_Lowpass_50 Hz ==
  error : Inport
  Dct2lowpass : sperte_lib/Dct2lowpass  f_den=140  b_den=0.5
      settings: SourceProductName=SPERTE project library
  Dctdoubleintegrator6 : S-Function  FunctionName=ddoubleint  Parameters=f_num, b_num, 0.001  SFunctionDeploymentMode=off  EnableBusSupport=off  mask(dctools){f_num=3.7, b_num=0.18}
      mask prompts: f_num "Zero [Hz]"; b_num "Damping [-]"
      mask help: This block implements a discrete time double-integrator filter with complex zero-pair.
      mask Display: disp('DCT double-integrator')
  Dctleadlag : sperte_lib/Dctleadlag  f_num=5.7  f_den=600
      settings: SourceProductName=SPERTE project library
  Dctnotch : sperte_lib/Dctnotch  f_num=60.6  b_num=0.001  f_den=85  b_den=0.68
      settings: SourceProductName=SPERTE project library
  Dctnotch2 : sperte_lib/Dctnotch  f_num=3.25  b_num=0.58  f_den=3.25  b_den=0.05
      settings: SourceProductName=SPERTE project library
  Gain2 : Gain  Gain=-0.998
  control signal : Outport
  wires:
  error/1 -> Gain2/1
  Gain2/1 -> Dctnotch/1
  Dctleadlag/1 -> Dctnotch2/1
  Dctnotch/1 -> Dctleadlag/1
  Dctnotch2/1 -> Dctdoubleintegrator6/1
  Dctdoubleintegrator6/1 -> Dct2lowpass/1
  Dct2lowpass/1 -> control signal/1

== system Reference_model_Control_Engineering/T9 Gain_Notch_60(Low second order)+3_LeadLag_Integrator_Lowpass_50 Hz1 ==
  error : Inport
  Dct2lowpass : sperte_lib/Dct2lowpass  f_den=140  b_den=0.5
      settings: SourceProductName=SPERTE project library
  Dctdoubleintegrator6 : S-Function  FunctionName=ddoubleint  Parameters=f_num, b_num, 0.001  SFunctionDeploymentMode=off  EnableBusSupport=off  mask(dctools){f_num=3.7, b_num=0.18}
      mask prompts: f_num "Zero [Hz]"; b_num "Damping [-]"
      mask help: This block implements a discrete time double-integrator filter with complex zero-pair.
      mask Display: disp('DCT double-integrator')
  Dctleadlag : sperte_lib/Dctleadlag  f_num=5.7  f_den=600
      settings: SourceProductName=SPERTE project library
  Dctnotch : sperte_lib/Dctnotch  f_num=60.6  b_num=0.001  f_den=85  b_den=0.68
      settings: SourceProductName=SPERTE project library
  Dctnotch2 : sperte_lib/Dctnotch  f_num=3.25  b_num=0.58  f_den=3.25  b_den=0.05
      settings: SourceProductName=SPERTE project library
  Gain2 : Gain  Gain=-0.998
  control signal : Outport
  wires:
  error/1 -> Gain2/1
  Gain2/1 -> Dctnotch/1
  Dctleadlag/1 -> Dctnotch2/1
  Dctnotch/1 -> Dctleadlag/1
  Dctnotch2/1 -> Dctdoubleintegrator6/1
  Dctdoubleintegrator6/1 -> Dct2lowpass/1
  Dct2lowpass/1 -> control signal/1

== system Reference_model_Control_Engineering/TA Gain_Notch_60(Second order)+3_LeadLag_Integrator_Lowpass_43.69_Medium_Noise Hz1 ==
  error : Inport
  Dct2lowpass : sperte_lib/Dct2lowpass  f_den=120  b_den=0.5
      settings: SourceProductName=SPERTE project library
  Dctintegrator : sperte_lib/Dctintegrator  f_num=5
      settings: SourceProductName=SPERTE project library
  Dctleadlag : sperte_lib/Dctleadlag  f_num=4.478  f_den=400
      settings: SourceProductName=SPERTE project library
  Dctnotch : sperte_lib/Dctnotch  f_num=60.6  b_num=0.015  f_den=105  b_den=0.3265
      settings: SourceProductName=SPERTE project library
  Dctnotch2 : sperte_lib/Dctnotch  f_num=3.25  b_num=0.5  f_den=3.25  b_den=0.025
      settings: SourceProductName=SPERTE project library
  Gain2 : Gain  Gain=-1.0049
  control signal : Outport
  wires:
  error/1 -> Gain2/1
  Gain2/1 -> Dctnotch/1
  Dctleadlag/1 -> Dctnotch2/1
  Dctnotch/1 -> Dctleadlag/1
  Dctnotch2/1 -> Dctintegrator/1
  Dctintegrator/1 -> Dct2lowpass/1
  Dct2lowpass/1 -> control signal/1

== system Reference_model_Control_Engineering/TB Gain_Notch_60(Second order notch)+3_LeadLag_DIntegrator_Lowpass_52.5_Medium_noise ==
  error : Inport
  Dct2lowpass : sperte_lib/Dct2lowpass  f_den=126.5  b_den=0.5
      settings: SourceProductName=SPERTE project library
  Dctdoubleintegrator6 : S-Function  FunctionName=ddoubleint  Parameters=f_num, b_num, 0.001  SFunctionDeploymentMode=off  EnableBusSupport=off  mask(dctools){f_num=4, b_num=0.4}
      mask prompts: f_num "Zero [Hz]"; b_num "Damping [-]"
      mask help: This block implements a discrete time double-integrator filter with complex zero-pair.
      mask Display: disp('DCT double-integrator')
  Dctleadlag : sperte_lib/Dctleadlag  f_num=5.35  f_den=350
      settings: SourceProductName=SPERTE project library
  Dctnotch : sperte_lib/Dctnotch  f_num=60.6  b_num=0.015  f_den=85  b_den=0.35
      settings: SourceProductName=SPERTE project library
  Dctnotch2 : sperte_lib/Dctnotch  f_num=3.25  b_num=0.5  f_den=3.25  b_den=0.001
      settings: SourceProductName=SPERTE project library
  Gain2 : Gain  Gain=-1.0049
  control signal : Outport
  wires:
  error/1 -> Gain2/1
  Gain2/1 -> Dctnotch/1
  Dctleadlag/1 -> Dctnotch2/1
  Dctnotch/1 -> Dctleadlag/1
  Dctnotch2/1 -> Dctdoubleintegrator6/1
  Dctdoubleintegrator6/1 -> Dct2lowpass/1
  Dct2lowpass/1 -> control signal/1

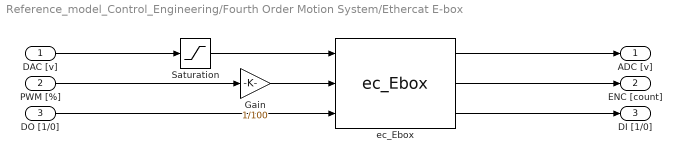
== system Reference_model_Control_Engineering/Fourth Order Motion System/Ethercat E-box ==
  DAC [v] : Inport
  PWM [%] : Inport  Port=2
  DO [1/0] : Inport  Port=3
  Gain : Gain  Gain=1/100
  Saturation : Saturate  UpperLimit=10  LowerLimit=-10
  ec_Ebox : S-Function  FunctionName=ec_Ebox  Parameters=link_id  SFunctionDeploymentMode=off  EnableBusSupport=off  mask{link_id=link_id}
      mask prompts: link_id "link_id >= 0"
      mask Display:
      | port_label('output',1,'ADC')
      | port_label('output',2,'ENC')
      | port_label('output',3,'DI')
      | port_label('input',1,'DAC')
      | port_label('input',2,'PWM')
      | port_label('input',3,'DO')
  ADC [v] : Outport
  ENC [count] : Outport  Port=2
  DI [1/0] : Outport  Port=3
  wires:
  Gain/1 -> ec_Ebox/2
  Saturation/1 -> ec_Ebox/1
  ec_Ebox/3 -> DI [1/0]/1
  ec_Ebox/1 -> ADC [v]/1
  ec_Ebox/2 -> ENC [count]/1
  DAC [v]/1 -> Saturation/1
  DO [1/0]/1 -> ec_Ebox/3
  PWM [%]/1 -> Gain/1

== system Reference_model_Control_Engineering/Fourth Order Motion System/Ethercat Supervisor ==
  note: Status, 0 = Operational, 1 = error
  S-Function : S-Function  FunctionName=ec_Supervisor  Parameters=portid,ectimeout  SFunctionDeploymentMode=off  EnableBusSupport=off
  Status : Outport
  wires:
  S-Function/1 -> Status/1

== matlab function Reference_model_Control_Engineering/Measurement Block/SPERTE_measurement_function ==
  data: u input double; status output uint8 size=[1]; trigger_manual input uint8 size=[1]; trigger_command input uint8 size=[1]; triggertype parameter uint8 size=[1]; N_samples input uint32 size=1
function status = perform_measurement(u, trigger_manual, trigger_command, triggertype, N_samples)

%% Persistent variables
persistent fileID NF busy NS

% Init parameters
if isempty(NF)
    NF = int16(0);
end
if isempty(NS)
    NS = uint32(0);
end
if isempty(fileID)
    fileID = 0;
end
if isempty(busy)
    busy = uint8(0);
end

%% Check the triggers
if ( (triggertype == 0 && trigger_manual == 1) || (triggertype == 1 && trigger_command == 1) || (triggertype == 2 && (trigger_command == 1 || trigger_manual == 1) ) )
    if busy == 1
        % We are already busy, nothing to do
    else
        % We should start a new one
        fileID = fopen(sprintf('measurement_%d.bin',NF),'w');  
        NF = NF + 1;
        busy = uint8(1);
        NS = uint32(0);
    end
end

% We have started a measurement
if busy == 1
    if NS < N_samples 
        % Here we write the sample, in single precision float
        fwrite(fileID,u,'single');
        NS = NS + uint32(1);
    else
       % We have N samples already, we are done
       fclose(fileID);
       busy = uint8(0);
       NS = uint32(0);
    end
      
end
    % Output state
    status = uint8(busy);
end

== matlab function Reference_model_Control_Engineering/MATLAB Function ==
  data: t input; a output; v output; p output
function [a,v,p] = fcn(t)
[p,v,a] = refGenSin(t,12);
